simulink model "mDataStoreBlocks"  (R2013b)
settings: Solver=FixedStepDiscrete  StartTime=0.0  StopTime=1  FixedStep=0.1  RelTol=1e-3
settings Model: Creator=hungdang  LastModifiedBy=hungdang
settings OptimizationCC: InlineParams=on  ActiveStateOutputEnumStorageType=Target Integer
settings DebuggingCC: InheritedTsInSrcMsg=none

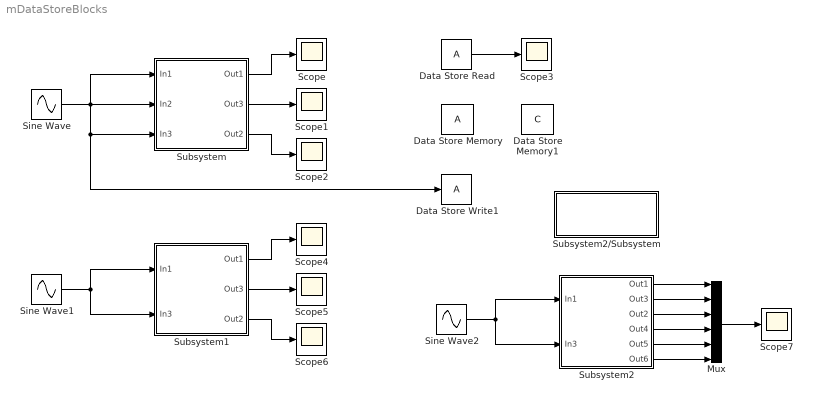
== system mDataStoreBlocks ==
  Data Store Memory : DataStoreMemory  ReadBeforeWriteMsg=warning  WriteAfterWriteMsg=warning  WriteAfterReadMsg=warning
  Data Store Memory1 : DataStoreMemory  DataStoreName=C  ReadBeforeWriteMsg=warning  WriteAfterWriteMsg=warning  WriteAfterReadMsg=warning
  Data Store Read : DataStoreRead
  Data Store Write1 : DataStoreWrite
  Mux : Mux  Inputs=6
  Scope{,1..7} (8 alike) : Scope
      Scope2 settings: SaveName=ScopeData2
      Scope3 settings: SaveName=ScopeData3
      Scope4 settings: SaveName=ScopeData4
      Scope5 settings: SaveName=ScopeData5
      Scope6 settings: SaveName=ScopeData6
      Scope7 settings: SaveName=ScopeData7
  Sine Wave : Sin  SampleTime=0.1
  Sine Wave1 : Sin  SineType=Sample based  SampleTime=0.1
  Sine Wave2 : Sin  SampleTime=0
  Subsystem : Subsystem  TreatAsAtomicUnit=on
  Subsystem1 : Subsystem  TreatAsAtomicUnit=on
  Subsystem2 : Subsystem  TreatAsAtomicUnit=on
      mask help: This is a simple mask.
  Subsystem2/Subsystem : Subsystem  TreatAsAtomicUnit=on
  wires:
  Sine Wave/1 -> Subsystem/1(In1), Data Store Write1/1, Subsystem/3(In3), Subsystem/2(In2)
  Subsystem/1(Out1) -> Scope/1
  Subsystem/2(Out3) -> Scope1/1
  Subsystem/3(Out2) -> Scope2/1
  Data Store Read/1 -> Scope3/1
  Sine Wave1/1 -> Subsystem1/1(In1), Subsystem1/2(In3)
  Subsystem1/1(Out1) -> Scope4/1
  Subsystem1/2(Out3) -> Scope5/1
  Subsystem1/3(Out2) -> Scope6/1
  Sine Wave2/1 -> Subsystem2/1(In1), Subsystem2/2(In3)
  Subsystem2/3(Out2) -> Mux/3
  Subsystem2/2(Out3) -> Mux/2
  Subsystem2/4(Out4) -> Mux/4
  Subsystem2/1(Out1) -> Mux/1
  Mux/1 -> Scope7/1
  Subsystem2/5(Out5) -> Mux/5
  Subsystem2/6(Out6) -> Mux/6

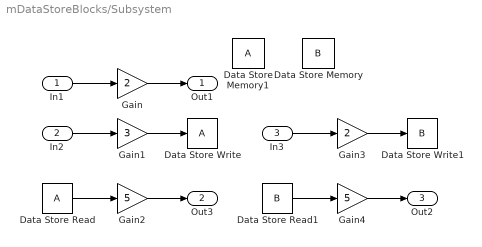
== system mDataStoreBlocks/Subsystem ==
  In1 : Inport
  In2 : Inport  Port=2
  In3 : Inport  Port=3
  Data Store Memory : DataStoreMemory  DataStoreName=B  ReadBeforeWriteMsg=warning  WriteAfterWriteMsg=warning  WriteAfterReadMsg=warning
  Data Store Memory1 : DataStoreMemory  ReadBeforeWriteMsg=warning  WriteAfterWriteMsg=warning  WriteAfterReadMsg=warning
  Data Store Read : DataStoreRead
  Data Store Read1 : DataStoreRead  DataStoreName=B
  Data Store Write : DataStoreWrite
  Data Store Write1 : DataStoreWrite  DataStoreName=B
  Gain : Gain  Gain=2
  Gain1 : Gain  Gain=3
  Gain2 : Gain  Gain=5
  Gain3 : Gain  Gain=2
  Gain4 : Gain  Gain=5
  Out1 : Outport
  Out3 : Outport  Port=2
  Out2 : Outport  Port=3
  wires:
  Gain/1 -> Out1/1
  In1/1 -> Gain/1
  Gain1/1 -> Data Store Write/1
  In2/1 -> Gain1/1
  Data Store Read/1 -> Gain2/1
  Gain2/1 -> Out3/1
  Gain3/1 -> Data Store Write1/1
  In3/1 -> Gain3/1
  Data Store Read1/1 -> Gain4/1
  Gain4/1 -> Out2/1

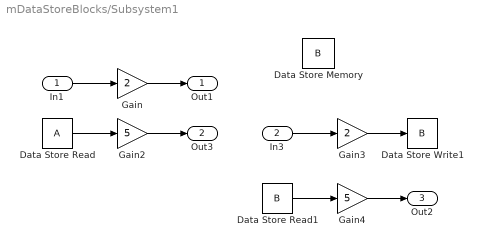
== system mDataStoreBlocks/Subsystem1 ==
  In1 : Inport
  In3 : Inport  Port=2
  Data Store Memory : DataStoreMemory  DataStoreName=B  ReadBeforeWriteMsg=warning  WriteAfterWriteMsg=warning  WriteAfterReadMsg=warning
  Data Store Read : DataStoreRead
  Data Store Read1 : DataStoreRead  DataStoreName=B
  Data Store Write1 : DataStoreWrite  DataStoreName=B
  Gain : Gain  Gain=2
  Gain2 : Gain  Gain=5
  Gain3 : Gain  Gain=2
  Gain4 : Gain  Gain=5
  Out1 : Outport
  Out3 : Outport  Port=2
  Out2 : Outport  Port=3
  wires:
  Gain/1 -> Out1/1
  In1/1 -> Gain/1
  Data Store Read/1 -> Gain2/1
  Gain2/1 -> Out3/1
  Gain3/1 -> Data Store Write1/1
  In3/1 -> Gain3/1
  Data Store Read1/1 -> Gain4/1
  Gain4/1 -> Out2/1

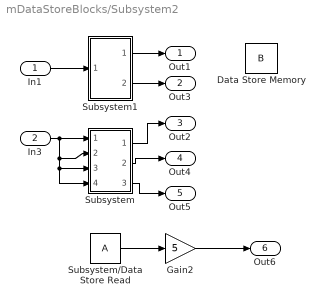
== system mDataStoreBlocks/Subsystem2 ==
  In1 : Inport
  In3 : Inport  Port=2
  Data Store Memory : DataStoreMemory  DataStoreName=B  ReadBeforeWriteMsg=warning  WriteAfterWriteMsg=warning  WriteAfterReadMsg=warning
  Gain2 : Gain  Gain=5
  Subsystem : Subsystem
  Subsystem/Data Store Read : DataStoreRead
  Subsystem1 : Subsystem
  Out1 : Outport
  Out3 : Outport  Port=2
  Out2 : Outport  Port=3
  Out4 : Outport  Port=4
  Out5 : Outport  Port=5
  Out6 : Outport  Port=6
  wires:
  In3/1 -> Subsystem/2(In1), Subsystem/4(In4), Subsystem/3(In2), Subsystem/1(In3)
  Subsystem/1(Out2) -> Out2/1
  In1/1 -> Subsystem1/1(In1)
  Subsystem1/1(Out1) -> Out1/1
  Subsystem1/2(Out3) -> Out3/1
  Subsystem/2(Out1) -> Out4/1
  Subsystem/3(Out3) -> Out5/1
  Gain2/1 -> Out6/1
  Subsystem/Data Store Read/1 -> Gain2/1

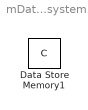
== system mDataStoreBlocks/Subsystem2//Subsystem ==
  Data Store Memory1 : DataStoreMemory  DataStoreName=C  ReadBeforeWriteMsg=warning  WriteAfterWriteMsg=warning  WriteAfterReadMsg=warning

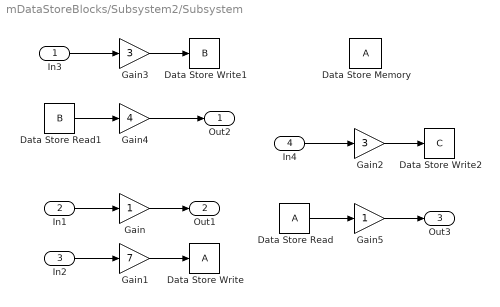
== system mDataStoreBlocks/Subsystem2/Subsystem ==
  In3 : Inport
  In1 : Inport  Port=2
  In2 : Inport  Port=3
  In4 : Inport  Port=4
  Data Store Memory : DataStoreMemory  ReadBeforeWriteMsg=warning  WriteAfterWriteMsg=warning  WriteAfterReadMsg=warning
  Data Store Read : DataStoreRead
  Data Store Read1 : DataStoreRead  DataStoreName=B
  Data Store Write : DataStoreWrite
  Data Store Write1 : DataStoreWrite  DataStoreName=B
  Data Store Write2 : DataStoreWrite  DataStoreName=C
  Gain : Gain
  Gain1 : Gain  Gain=7
  Gain2 : Gain  Gain=3
  Gain3 : Gain  Gain=3
  Gain4 : Gain  Gain=4
  Gain5 : Gain
  Out2 : Outport
  Out1 : Outport  Port=2
  Out3 : Outport  Port=3
  wires:
  In3/1 -> Gain3/1
  Gain4/1 -> Out2/1
  Data Store Read1/1 -> Gain4/1
  Gain3/1 -> Data Store Write1/1
  Gain/1 -> Out1/1
  In1/1 -> Gain/1
  Gain1/1 -> Data Store Write/1
  In2/1 -> Gain1/1
  Data Store Read/1 -> Gain5/1
  Gain5/1 -> Out3/1
  In4/1 -> Gain2/1
  Gain2/1 -> Data Store Write2/1

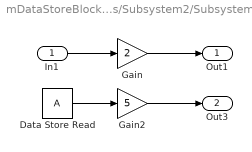
== system mDataStoreBlocks/Subsystem2/Subsystem1 ==
  In1 : Inport
  Data Store Read : DataStoreRead
  Gain : Gain  Gain=2
  Gain2 : Gain  Gain=5
  Out1 : Outport
  Out3 : Outport  Port=2
  wires:
  Gain2/1 -> Out3/1
  In1/1 -> Gain/1
  Data Store Read/1 -> Gain2/1
  Gain/1 -> Out1/1
